simulink model "untitled222_SG"  (Simulink 7.1)
settings: Solver=ode45  StartTime=0.0  StopTime=600  RelTol=1e-3
settings Model: Creator=Admin  LastModifiedBy=aast

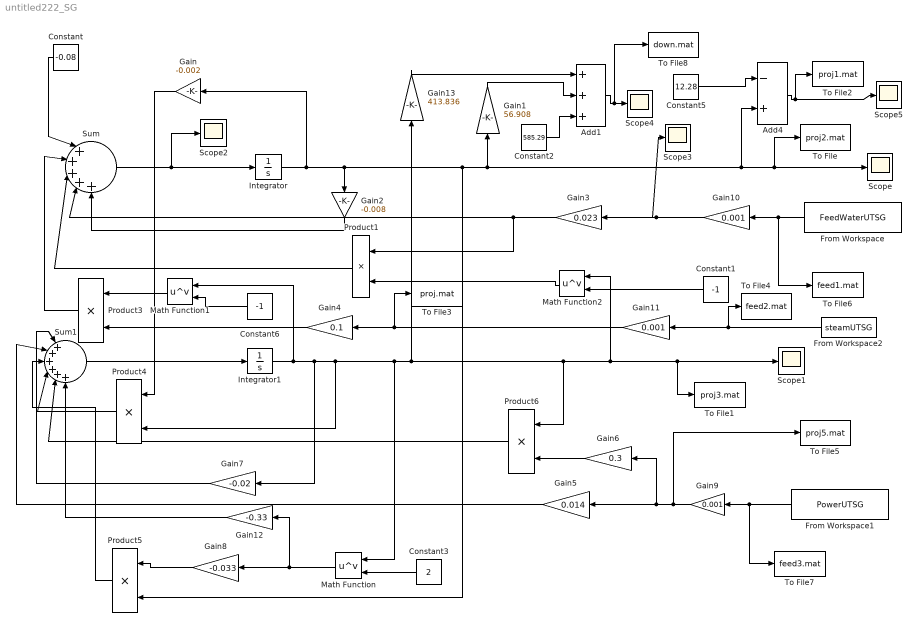
== system untitled222_SG ==
  Add1 : Sum  Inputs=+++  OutDataType=sfix(16)  OutScaling=2^-10
  Add4 : Sum  Inputs=-+  OutDataType=sfix(16)  OutScaling=2^-10
  Constant : Constant  Orientation=left  Value=-0.08  OutDataType=sfix(16)  OutScaling=2^0
  Constant1 : Constant  Orientation=left  Value=-1  OutDataType=sfix(16)  OutScaling=2^0
  Constant2 : Constant  Value=585.29  OutDataType=sfix(16)  OutScaling=2^0
  Constant3 : Constant  Orientation=left  Value=2  OutDataType=sfix(16)  OutScaling=2^0
  Constant5 : Constant  Value=12.28  OutDataType=sfix(16)  OutScaling=2^0
  Constant6 : Constant  Orientation=left  Value=-1  OutDataType=sfix(16)  OutScaling=2^0
  From Workspace : FromWorkspace  Orientation=left  VariableName=FeedWaterUTSG  SampleTime=0
  From Workspace1 : FromWorkspace  Orientation=left  VariableName=PowerUTSG  SampleTime=0
  From Workspace2 : FromWorkspace  Orientation=left  VariableName=steamUTSG  SampleTime=0
  Gain : Gain  Orientation=left  Gain=-0.002  ParameterDataType=sfix(16)  ParameterScaling=2^0  OutDataType=sfix(16)  OutScaling=2^0
  Gain1 : Gain  Orientation=up  Gain=56.908  ParameterDataType=sfix(16)  ParameterScaling=2^0  OutDataType=sfix(16)  OutScaling=2^0
  Gain10 : Gain  Orientation=left  Gain=0.001  ParameterDataType=sfix(16)  ParameterScaling=2^0  OutDataType=sfix(16)  OutScaling=2^0
  Gain11 : Gain  Orientation=left  Gain=0.001  ParameterDataType=sfix(16)  ParameterScaling=2^0  OutDataType=sfix(16)  OutScaling=2^0
  Gain12 : Gain  Orientation=left  Gain=-0.33  ParameterDataType=sfix(16)  ParameterScaling=2^0  OutDataType=sfix(16)  OutScaling=2^0
  Gain13 : Gain  Orientation=up  Gain=413.836  ParameterDataType=sfix(16)  ParameterScaling=2^0  OutDataType=sfix(16)  OutScaling=2^0
  Gain2 : Gain  Orientation=down  Gain=-0.008  ParameterDataType=sfix(16)  ParameterScaling=2^0  OutDataType=sfix(16)  OutScaling=2^0
  Gain3 : Gain  Orientation=left  Gain=0.023  ParameterDataType=sfix(16)  ParameterScaling=2^0  OutDataType=sfix(16)  OutScaling=2^0
  Gain4 : Gain  Orientation=left  Gain=0.1  ParameterDataType=sfix(16)  ParameterScaling=2^0  OutDataType=sfix(16)  OutScaling=2^0
  Gain5 : Gain  Orientation=left  Gain=0.014  ParameterDataType=sfix(16)  ParameterScaling=2^0  OutDataType=sfix(16)  OutScaling=2^0
  Gain6 : Gain  Orientation=left  Gain=0.3  ParameterDataType=sfix(16)  ParameterScaling=2^0  OutDataType=sfix(16)  OutScaling=2^0
  Gain7 : Gain  Orientation=left  Gain=-0.02  ParameterDataType=sfix(16)  ParameterScaling=2^0  OutDataType=sfix(16)  OutScaling=2^0
  Gain8 : Gain  Orientation=left  Gain=-0.033  ParameterDataType=sfix(16)  ParameterScaling=2^0  OutDataType=sfix(16)  OutScaling=2^0
  Gain9 : Gain  Orientation=left  Gain=0.001  ParameterDataType=sfix(16)  ParameterScaling=2^0  OutDataType=sfix(16)  OutScaling=2^0
  Integrator : Integrator  InitialCondition=12.28
  Integrator1 : Integrator  InitialCondition=0.28
  Math Function : Math  Orientation=left  Operator=pow  OutDataType=sfix(16)  OutScaling=2^0  SaturateOnIntegerOverflow=on
  Math Function1 : Math  Orientation=left  Operator=pow  OutDataType=sfix(16)  OutScaling=2^0  SaturateOnIntegerOverflow=on
  Math Function2 : Math  Orientation=left  Operator=pow  OutDataType=sfix(16)  OutScaling=2^0  SaturateOnIntegerOverflow=on
  Product{1,3..6} (5 alike) : Product  Orientation=left  OutDataType=sfix(16)  OutScaling=2^0  RndMeth=Zero
  Scope{,1..5} (6 alike) : Scope
      Scope settings: TimeRange=600  YMin=0  YMax=14
      Scope1 settings: TimeRange=600  YMin=0.05  YMax=0.3
      Scope2 settings: TimeRange=600  YMin=-2  YMax=14  SaveName=ScopeData2
      Scope3 settings: TimeRange=600  YMin=-2  YMax=14  SaveName=ScopeData3
      Scope4 settings: TimeRange=6  YMin=1424  YMax=1432  SaveName=ScopeData4
      Scope5 settings: TimeRange=600  YMin=-1  YMax=6  SaveName=ScopeData5
  Sum : Sum  Inputs=|+++++  OutDataType=sfix(16)  OutScaling=2^0
  Sum1 : Sum  Inputs=|++++++  OutDataType=sfix(16)  OutScaling=2^0
  To File : ToFile  Filename=proj2.mat  MatrixName=vv
  To File1 : ToFile  Filename=proj3.mat  MatrixName=vv
  To File2 : ToFile  Filename=proj1.mat  MatrixName=vv
  To File3 : ToFile  Filename=proj.mat  MatrixName=vv
  To File4 : ToFile  Filename=feed2.mat  MatrixName=vv
  To File5 : ToFile  Filename=proj5.mat  MatrixName=vv
  To File6 : ToFile  Filename=feed1.mat  MatrixName=vv
  To File7 : ToFile  Filename=feed3.mat  MatrixName=vv
  To File8 : ToFile  Filename=down.mat  MatrixName=vv
  wires:
  Sum/1 -> Integrator/1, Scope2/1
  Integrator1/1 -> Math Function1/1, Gain7/1, Math Function/1, Math Function2/1, Scope1/1, To File1/1, Product6/1, Gain13/1, Product4/2
  Gain5/1 -> Sum1/2
  Math Function/1 -> Gain8/1, Gain12/1
  Integrator/1 -> Gain2/1, Product5/2, Add4/2, Scope/1, To File/1, Gain1/1, Gain/1
  From Workspace1/1 -> Gain9/1, To File7/1
  From Workspace/1 -> Gain10/1, To File6/1
  Gain10/1 -> Gain3/1, Scope3/1
  From Workspace2/1 -> Gain11/1, To File4/1
  Gain11/1 -> Gain4/1, To File3/1
  Constant5/1 -> Add4/1
  Add4/1 -> Scope5/1, To File2/1
  Gain4/1 -> Product3/2
  Math Function1/1 -> Product3/1
  Product3/1 -> Sum/2
  Constant3/1 -> Math Function/2
  Constant6/1 -> Math Function1/2
  Constant1/1 -> Math Function2/2
  Gain/1 -> Product4/1
  Product1/1 -> Sum/3
  Product4/1 -> Sum1/4
  Gain8/1 -> Product5/1
  Product5/1 -> Sum1/3
  Gain9/1 -> Gain5/1, Gain6/1, To File5/1
  Gain6/1 -> Product6/2
  Product6/1 -> Sum1/5
  Gain7/1 -> Sum1/1
  Gain12/1 -> Sum1/6
  Constant/1 -> Sum/1
  Gain2/1 -> Sum/5
  Math Function2/1 -> Product1/2
  Gain3/1 -> Sum/4, Product1/1
  Sum1/1 -> Integrator1/1
  Gain1/1 -> Add1/2
  Gain13/1 -> Add1/1
  Constant2/1 -> Add1/3
  Add1/1 -> Scope4/1, To File8/1
